simulink model "simple"  (R2020b)
settings: Solver=VariableStepAuto  StartTime=0.0  StopTime=Tf  RelTol=1e-3
values from neighbouring files (symbols this model uses):
  map = binaryOccupancyMap(maze, res)    [Run_Sim_LC.m]    (also in lidarPlanner.m = binaryOccupancyMap(                 [mapXLimits(2)-mapXLimit)
  N = size(waypoints, 1)    [interpolate_leg_waypoints.m]
  startPose = [2 2 0]    [Run_Sim_LC.m]
  Ts = 0.01    [Run_Sim_LC.m]
  waypoints = zeros(N, 4)    [get_leg_waypoints.m]    (also in leg_waypoints.m = linspace(start_config, goal_config, N); lidarPlanner.m = refpath.States(:,1:2))
undefined symbols (not defined in the file or in its folder): Discrete, Time, X, Y, Z
libraries: sm_lib x12, nesl_utility x3, hexapod x2, robotics_pg_exp_pack x2, ctrlSharedLib x1, robotalgslib x1
settings Model: Creator=fciriell  LastModifiedBy=zach
settings ExplorerConfigSet: InternalSimMechanicsExplorerSettings="<ExplorerConfiguration><canonicalview>default</canonicalview><AnimationSetting><BasePlaybackSpeed>1.0</BasePlaybackSpeed><PlaybackSpeedFactor>1.0</PlaybackSpeedFactor></AnimationSetting><TilePanel><TileInfo><Tiles Columns=\"1\" Count=\"2\" Rows=\"2\"><Column Weight=\"1\"/><Row Weight=\"0.4993\"/><Row Weight=\"0.5007\"/><Tile Height=\"1\" Width=\"1\" X=\"0\" Y=\"0\"/><Tile Height=\"1\" Width=\"1\" X=\"0\" Y=\"1\"/></Tiles></TileInfo><SceneInfo><SceneViewer><BGColor><R>1</R><G>1</G><B>1</B></BGColor><Camera><DoPerspective>on</DoPerspective><Position><X>-4.35147948962821829e-06</X><Y>-4.89869399804638128</Y><Z>0.176731420553238427</Z></Position><Center><X>-4.35147948962821829e-06</X><Y>-1.26250265135058726</Y><Z>0.176731420553238427</Z></Center><Up><X>0</X><Y>-0</Y><Z>1</Z></Up><ViewLimDist>1</ViewLimDist><YLim>0.466307658154998583</YLim><XLim>1.59125758717581123</XLim></Camera></SceneViewer><SceneViewer><BGColor><R>1</R><G>1</G><B>1</B></BGColor><Camera><DoPerspective>off</DoPerspective><Position><X>-5.9945065800093289e-08</X><Y>-3.21515629578642415</Y><Z>0.0606596897011122405</Z></Position><Center><X>-5.9945065800093289e-08</X><Y>-1.26250000733898382</Y><Z>0.0606596897011122405</Z></Center><Up><X>-0</X><Y>0</Y><Z>1</Z></Up><ViewLimDist>1</ViewLimDist><YLim>0.993270539045333911</YLim><XLim>3.37947076894122489</XLim></Camera></SceneViewer></SceneInfo></TilePanel><MechEditorPanel><Cameras><Camera><Id>Camera1</Id><Value><Name>Camera1</Name><NativeCamera><PositionTrackingFeature>camera.F</PositionTrackingFeature><CenterTrackingFeature>One_link_chain_dynamic.to_WF</CenterTrackingFeature><UpVectorTrackingFeature>camera.F</UpVectorTrackingFeature><CenterTrackingOrigin>on</CenterTrackingOrigin><UpVectorTrackingDirection>+Z</UpVectorTrackingDirection></NativeCamera></Value></Camera></Cameras><GfxPanelCameraMap><MapElement CameraMLId=\"Camera1\" GfxPanelIndex=\"0\"/></GfxPanelCameraMap><VideoCreator><PlaybackSpeedRatio>1.0</PlaybackSpeedRatio><FrameRate>30</FrameRate><VideoFormat>Motion JPEG AVI</VideoFormat><FrameSize>auto</FrameSize></VideoCreator></MechEditorPanel></ExplorerConfiguration>"

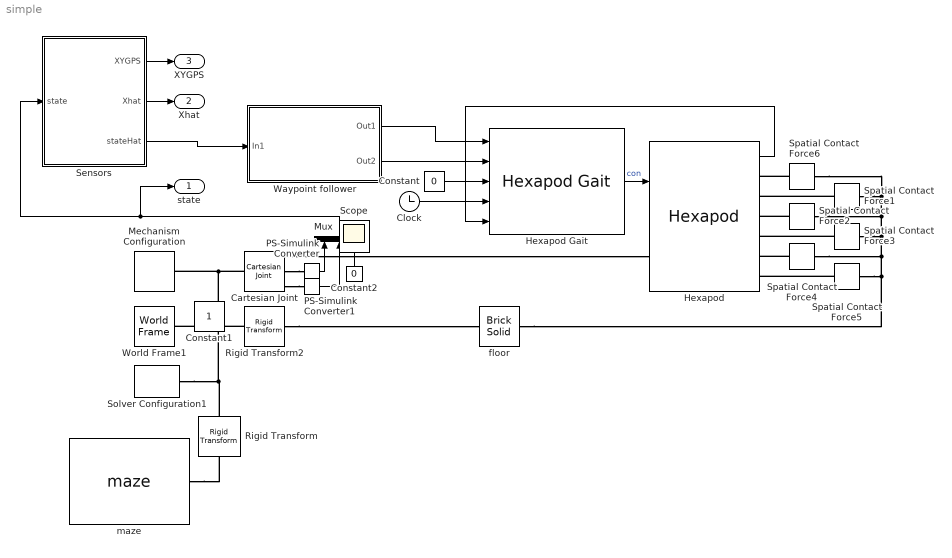
== system simple ==
  Cartesian Joint : sm_lib/Joints/Cartesian Joint  JointMode=Normal  SenseConstraintForce=off  SenseConstraintForceX=off  SenseConstraintForceY=off  SenseConstraintForceZ=off  SenseConstraintTorque=off  SenseConstraintTorqueX=off  SenseConstraintTorqueY=off  SenseConstraintTorqueZ=off  SenseTotalForce=off  SenseTotalForceX=off  SenseTotalForceY=off  SenseTotalForceZ=off  SenseTotalTorque=off  SenseTotalTorqueX=off  SenseTotalTorqueY=off  SenseTotalTorqueZ=off  CompositeWrenchDir=FollowerOnBase  CompositeWrenchFrame=BaseFrame  PxEquilibriumPosition=0  PxEquilibriumPositionUnits=m  PxSpringStiffness=0  PxSpringStiffnessUnits=N/m  PxDampingCoefficient=0  PxDampingCoefficientUnits=N/(m/s)  PxTorqueActuationMode=NoTorque  PxMotionActuationMode=ComputedMotion  PxSensePosition=on  PxSenseVelocity=off  PxSenseAcceleration=off  PxSenseTorqueForce=off  PxSenseLowerLimitTorqueForce=off  PxSenseUpperLimitTorqueForce=off  PxLowerLimitSpecify=off  PxLowerLimitBound=-1  PxLowerLimitBoundUnits=m  PxLowerLimitStiffness=1e6  PxLowerLimitStiffnessUnits=N/m  PxLowerLimitDamping=1e3  PxLowerLimitDampingUnits=N/(m/s)  PxLowerLimitTransitionRegionWidth=1e-4  PxLowerLimitTransitionRegionWidthUnits=m  PxUpperLimitSpecify=off  PxUpperLimitBound=1  PxUpperLimitBoundUnits=m  PxUpperLimitStiffness=1e6  PxUpperLimitStiffnessUnits=N/m  PxUpperLimitDamping=1e3  PxUpperLimitDampingUnits=N/(m/s)  PxUpperLimitTransitionRegionWidth=1e-4  PxUpperLimitTransitionRegionWidthUnits=m  PxPositionTargetSpecify=on  PxPositionTargetPriority=High  PxPositionTargetValue=startPose(1)  PxPositionTargetValueUnits=m  PxVelocityTargetSpecify=off  PxVelocityTargetPriority=High  PxVelocityTargetValue=0  PxVelocityTargetValueUnits=m/s  PyEquilibriumPosition=0  PyEquilibriumPositionUnits=m  PySpringStiffness=0  PySpringStiffnessUnits=N/m  PyDampingCoefficient=0  PyDampingCoefficientUnits=N/(m/s)  PyTorqueActuationMode=NoTorque  PyMotionActuationMode=ComputedMotion  PySensePosition=on  PySenseVelocity=off  PySenseAcceleration=off  PySenseTorqueForce=off  PySenseLowerLimitTorqueForce=off  PySenseUpperLimitTorqueForce=off  PyLowerLimitSpecify=off  PyLowerLimitBound=-1  PyLowerLimitBoundUnits=m  PyLowerLimitStiffness=1e6  PyLowerLimitStiffnessUnits=N/m  PyLowerLimitDamping=1e3  PyLowerLimitDampingUnits=N/(m/s)  PyLowerLimitTransitionRegionWidth=1e-4  PyLowerLimitTransitionRegionWidthUnits=m  PyUpperLimitSpecify=off  PyUpperLimitBound=1  PyUpperLimitBoundUnits=m  PyUpperLimitStiffness=1e6  PyUpperLimitStiffnessUnits=N/m  PyUpperLimitDamping=1e3  PyUpperLimitDampingUnits=N/(m/s)  PyUpperLimitTransitionRegionWidth=1e-4  PyUpperLimitTransitionRegionWidthUnits=m  PyPositionTargetSpecify=on  PyPositionTargetPriority=High  PyPositionTargetValue=startPose(2)  PyPositionTargetValueUnits=m  PyVelocityTargetSpecify=off  PyVelocityTargetPriority=High  PyVelocityTargetValue=0  PyVelocityTargetValueUnits=m/s  PzEquilibriumPosition=0  PzEquilibriumPositionUnits=m  PzSpringStiffness=0  PzSpringStiffnessUnits=N/m  PzDampingCoefficient=0  PzDampingCoefficientUnits=N/(m/s)  PzTorqueActuationMode=NoTorque  PzMotionActuationMode=ComputedMotion  PzSensePosition=off  PzSenseVelocity=off  PzSenseAcceleration=off  PzSenseTorqueForce=off  PzSenseLowerLimitTorqueForce=off  PzSenseUpperLimitTorqueForce=off  PzLowerLimitSpecify=off  PzLowerLimitBound=-1  PzLowerLimitBoundUnits=m  PzLowerLimitStiffness=1e6  PzLowerLimitStiffnessUnits=N/m  PzLowerLimitDamping=1e3  PzLowerLimitDampingUnits=N/(m/s)  PzLowerLimitTransitionRegionWidth=1e-4  PzLowerLimitTransitionRegionWidthUnits=m  PzUpperLimitSpecify=off  PzUpperLimitBound=1  PzUpperLimitBoundUnits=m  PzUpperLimitStiffness=1e6  PzUpperLimitStiffnessUnits=N/m  PzUpperLimitDamping=1e3  PzUpperLimitDampingUnits=N/(m/s)  PzUpperLimitTransitionRegionWidth=1e-4  PzUpperLimitTransitionRegionWidthUnits=m  PzPositionTargetSpecify=on  PzPositionTargetPriority=High  PzPositionTargetValue=0.35  PzPositionTargetValueUnits=m  PzVelocityTargetSpecify=off  PzVelocityTargetPriority=High  PzVelocityTargetValue=0  PzVelocityTargetValueUnits=m/s
  Clock : Clock
  Constant : Constant  Value=0  SampleTime=-1
  Constant2 : Constant  Value=0
  Hexapod : hexapod/Hexapod  leg_initial_config=[0; -pi/8; 5*pi/8]  leg_length_1=0.1  leg_length_2=0.4  leg_length_3=0.4  leg_radius=0.04  leg_mass_1=0.1  leg_mass_2=0.3  leg_mass_3=0.3  pos_kp=[80; 80; 80]  pos_ki=[0; 0; 0]  pos_kd=[10; 10; 10]  body_radius=0.3  body_mass=0.2
  Hexapod Gait : hexapod/Hexapod Gait  beta=0.55  T=0.6  contact_start_config=[0; -pi/8; 5*pi/8]  lifted_mid_theta2=-pi/4  lifted_mid_theta3=3*pi/4  body_radius=0.3  leg_length_1=0.1  leg_length_2=0.4  leg_length_3=0.4
  Mechanism Configuration : sm_lib/Utilities/Mechanism Configuration  UniformGravity=Constant  GravityVector=[0 0 -9.80665]  GravityVectorUnits=m/s^2  GravityUnits=m/s^2  LinearizationDelta=0.001  JointModeTransitionNonlinearIterations=2
  Mux : Mux  Inputs=3
  PS-Simulink Converter : nesl_utility/PS-Simulink Converter  PhysicalDomain=network_engine_domain  SubClassName=ps_output  LeftPortType=input  RightPortType=output  PseudoPeriodic=off  Frequencies=[]  Unit=inherit  AffineConversion=off
  PS-Simulink Converter1 : nesl_utility/PS-Simulink Converter  PhysicalDomain=network_engine_domain  SubClassName=ps_output  LeftPortType=input  RightPortType=output  PseudoPeriodic=off  Frequencies=[]  Unit=inherit  AffineConversion=off
  Rigid Transform : sm_lib/Frames and Transforms/Rigid Transform  TranslationMethod=StandardAxis  TranslationStandardOffset=0.01  TranslationLengthUnit=m  TranslationStandardAxis=-Z  TranslationCartesianOffset=[0 0 0]  TranslationROffset=0  TranslationROffsetUnits=m  TranslationZOffset=0  TranslationZOffsetUnits=m  TranslationThetaOffset=0  TranslationThetaOffsetUnits=deg  RotationMethod=None  RotationAngleUnits=deg  RotationStandardAxis=+Z  RotationAngle=0.0  RotationArbitraryAxis=[0 0 1]  FollAlignAxisA=+X  BaseAlignAxisA=+Y  FollAlignAxisB=+Y  BaseAlignAxisB=+Z  RotationSequenceAxes=FollowerAxes  RotationSequence=XYX  RotationSequenceAngles=[0 0 0]  RotationSequenceAnglesUnits=deg  RotationMatrix=[1 0 0; 0 1 0; 0 0 1]
  Rigid Transform2 : sm_lib/Frames and Transforms/Rigid Transform  TranslationMethod=Cartesian  TranslationStandardOffset=0  TranslationLengthUnit=m  TranslationStandardAxis=+Z  TranslationCartesianOffset=[(map.XWorldLimits(1)+map.XWorldLimits(2))/2 (map.YWorldLimits(1)+map.YWorldLimits(2))/2 0]  TranslationROffset=0  TranslationROffsetUnits=m  TranslationZOffset=0  TranslationZOffsetUnits=m  TranslationThetaOffset=0  TranslationThetaOffsetUnits=deg  RotationMethod=None  RotationAngleUnits=deg  RotationStandardAxis=+Z  RotationAngle=0.0  RotationArbitraryAxis=[0 0 1]  FollAlignAxisA=+X  BaseAlignAxisA=+Y  FollAlignAxisB=+Y  BaseAlignAxisB=+Z  RotationSequenceAxes=FollowerAxes  RotationSequence=XYX  RotationSequenceAngles=[0 0 0]  RotationSequenceAnglesUnits=deg  RotationMatrix=[1 0 0; 0 1 0; 0 0 1]
  Sensors : Subsystem
  Solver Configuration1 : nesl_utility/Solver Configuration  PhysicalDomain=network_engine_domain  SubClassName=solver  LeftPortType=input  RightPortType=generic  Tones=[]  Harmonics=[]  SimulateNoise=off  Profile=off  UseLocalSampling=off  EnableSwitchedLinearOptims=on  FrequencyDomain=off  UseCCode=off  RelTol=0.001  AbsTol=1e-06  MinStep=1e-09  ToWorkspace=off  RevertToSquareIcSolve=off  NumHomotopyIterations=100  PhasorMode=off  PhasorModeNumHarmonics=1  DoDC=off  ResidualTolerance=1e-09  UseLocalSolver=off  LocalSolverChoice=NE_BACKWARD_EULER_ADVANCER  LocalSolverSampleTime=0.001  DoFixedCost=off  MaxNonlinIter=3  MaxModeIter=2  ComputeImpulses=off  ImpulseIterations=2  LinearAlgebra=auto  EquationFormulation=NE_TIME_EF  DelaysMemoryBudget=1024  AutomaticFiltering=on  FilteringTimeConstant=0.001  PartitionStorageMethod=AS_NEEDED  PartitionMemoryBudget=1024  PartitionMethod=ROBUST
  Spatial Contact Force{1..6} (6 alike) : sm_lib/Forces and Torques/Spatial Contact Force  CoefficientOfDynamicFriction=0.3  CoefficientOfStaticFriction=0.9  NormalDamping=1e3  NormalDampingUnits=N/(m/s)  NormalStiffness=1e6  NormalStiffnessUnits=N/m  FrictionalCriticalVelocity=1e-3  FrictionalCriticalVelocityUnits=m/s  ZeroCrossDetectContactStartAndEnd=off  SenseFrictionalForceMagnitude=off  SenseNormalForceMagnitude=off  SenseSeparationDistance=off  NormalTransitionRegionWidth=1e-4  NormalTransitionRegionWidthUnits=m  FrictionType=SmoothStickSlip
  Waypoint follower : Subsystem
  World Frame1 : sm_lib/Frames and Transforms/World Frame
  floor : sm_lib/Body Elements/Brick Solid  GraphicAmbientColor=[0.15 0.15 0.15 1.0]  BasedOnType=Density  BrickDimensions=[(map.XWorldLimits(2)-map.XWorldLimits(1)) (map.YWorldLimits(2)-map.YWorldLimits(1)) 0.5]  BrickDimensionUnits=m  CenterOfMass=[0 0 0]  CenterOfMassUnits=m  GraphicDiffuseColor=[0.5 0.5 0.5]  Density=1000  DensityUnits=kg/m^3  DoExposeReferenceFrame=off  GraphicEmissiveColor=[0.0 0.0 0.0 1.0]  ExportEntireGeometry=on  SerializedFrames=<Frames><Frame><Id>Frame1</Id><Value><Name>TF</Name><Origin><Source>GeometricFeature</Source><FeatureName>+z surface</FeatureName></Origin><PrimaryAxis><DefinedDirection>+Z</DefinedDirection><Source>ReferenceFrame</Source><SourceDirection>+Z</SourceDirection><FeatureName></FeatureName></PrimaryAxis><SecondaryAxis><DefinedDirection>+X</DefinedDirection><Source>ReferenceFrame</Source><SourceDirection>+X</SourceDirection><FeatureName></FeatureName></SecondaryAxis></Value></Frame></Frames>  MarkerShape=Sphere  MarkerSize=10  GraphicType=FromGeometry  InertiaType=CalculateFromGeometry  Mass=1  MassUnits=kg  MomentsOfInertia=[1 1 1]  MomentsOfInertiaUnits=kg*m^2  GraphicOpacity=0.5  ProductsOfInertia=[0 0 0]  ProductsOfInertiaUnits=kg*m^2  GraphicShininess=75  GraphicSpecularColor=[0.5 0.5 0.5 1.0]  GraphicVisPropType=SimpleVisualProperties
  maze : robotics_pg_exp_pack/Environments & Sensors/Simscape Multibody Environments/maze  map=maze  wall_height=0.5  resolution=res  branching=branching
      settings: SourceProductName=Robotics Playground Expansion Pack
  state : Outport
  Xhat : Outport  Port=2
  XYGPS : Outport  Port=3
  Constant1 : Constant  IOType=siggen
  Scope : Scope
  wires:
  Hexapod Gait/1 -> Hexapod/1  "con"
  Hexapod/1 -> Hexapod Gait/5
  Constant/1 -> Hexapod Gait/3
  Clock/1 -> Hexapod Gait/4
  Mux/1 -> state/1, Sensors/1(state)
  Sensors/1(XYGPS) -> XYGPS/1
  Sensors/2(Xhat) -> Xhat/1
  Sensors/3(stateHat) -> Waypoint follower/1(In1)
  Waypoint follower/1(Out1) -> Hexapod Gait/1
  Waypoint follower/2(Out2) -> Hexapod Gait/2
  PS-Simulink Converter1/1 -> Mux/2
  PS-Simulink Converter/1 -> Mux/1
  Constant2/1 -> Mux/3
  connections:
  Cartesian Joint/RConn1 -- Hexapod/LConn1
  floor/RConn1 -- Spatial Contact Force5/LConn1 -- Spatial Contact Force4/LConn1 -- Spatial Contact Force3/LConn1 -- Spatial Contact Force2/LConn1 -- Spatial Contact Force1/LConn1 -- Spatial Contact Force6/LConn1
  Spatial Contact Force6/RConn1 -- Hexapod/RConn1
  Spatial Contact Force1/RConn1 -- Hexapod/RConn2
  Spatial Contact Force3/RConn1 -- Hexapod/RConn4
  Spatial Contact Force5/RConn1 -- Hexapod/RConn6
  Spatial Contact Force4/RConn1 -- Hexapod/RConn5
  Spatial Contact Force2/RConn1 -- Hexapod/RConn3
  Rigid Transform2/RConn1 -- floor/LConn1
  Solver Configuration1/RConn1 -- Rigid Transform/LConn1 -- Rigid Transform2/LConn1 -- Cartesian Joint/LConn1 -- Mechanism Configuration/RConn1 -- World Frame1/RConn1
  maze/RConn1 -- Rigid Transform/RConn1
  Cartesian Joint/RConn2 -- PS-Simulink Converter/LConn1
  Cartesian Joint/RConn3 -- PS-Simulink Converter1/LConn1

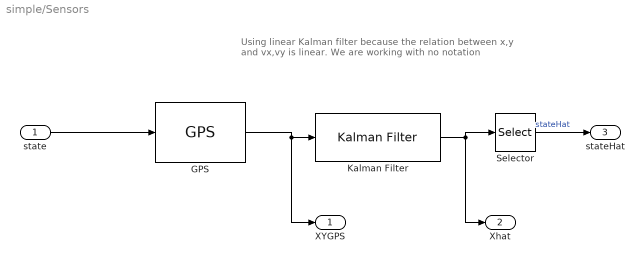
== system simple/Sensors ==
  note: Using linear Kalman filter because the relation between x,y and vx,vy is linear. We are working with no notation
  state : Inport
  "GPS " : robotics_pg_exp_pack/Environments & Sensors/GPS  xNoisePower=0.05  yNoisePower=0.05  Ts=Ts
      settings: SourceProductName=Robotics Playground Expansion Pack
  "Kalman Filter " : ctrlSharedLib/Kalman Filter  TimeDomain=Discrete-Time  UseCurrentEstimator=on  ModelSource=Individual A, B, C, D matrices  ModelSourceVariable=sys  A=[1 0 Ts 0; 0 1 0 Ts; 0 0 1 0; 0 0 0 1]  B=[0 0; 0 0; 1 0; 0 1]  C=[1 0 0 0; 0 1 0 0]  D=zeros(2)  NumberOfStates=2  NumberOfInputs=2  NumberOfOutputs=2  InitialEstimateSource=Dialog  X0=[startPose(1) startPose(2) 0 0]  P0=1e-3  UseK=off  UseGH=on  NumberOfProcessNoiseInputs=2  G=[Ts/2 0; 0 Ts/2; 1 0; 0 1]  TimeInvariantG=on  H=0  TimeInvariantH=on  Q=0.12  TimeInvariantQ=on  R=0.08  TimeInvariantR=on  N=0  TimeInvariantN=on  AddInputPort=off  AddEnablePort=off  OutputEstimatedY=off  OutputP=off  Ts=Ts
  Selector : Selector  InputPortWidth=4  IndexOptions=Index vector (dialog)  Indices=[1 2]  OutputSizes=1
  XYGPS : Outport
  Xhat : Outport  Port=2
  stateHat : Outport  Port=3
  wires:
  "GPS "/1 -> XYGPS/1, "Kalman Filter "/1
  Selector/1 -> stateHat/1  "stateHat"
  "Kalman Filter "/1 -> Selector/1, Xhat/1
  state/1 -> "GPS "/1

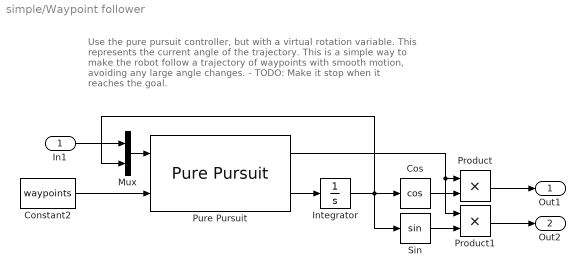
== system simple/Waypoint follower ==
  note: Use the pure pursuit controller, but with a virtual rotation variable.
      | This represents the current angle of the trajectory. This is a simple
      | way to make the robot follow a trajectory of waypoints with smooth
      | motion, avoiding any large angle changes.
      | - TODO: Make it stop when it reaches the goal.
  In1 : Inport
  Constant2 : Constant  Value=waypoints
  Cos : Trigonometry  Operator=cos
  Integrator : Integrator  InitialCondition=atan2(waypoints(2,2)-startPose(2), waypoints(1,2)-startPose(1))  WrapState=on
  Mux : Mux  Inputs=2
  Product : Product
  Product1 : Product
  Pure Pursuit : robotalgslib/Pure Pursuit  DesiredLinearVelocity=0.8  MaxAngularVelocity=3.14  LookaheadDistance=1.0  TargetDirPort=off  SimulateUsing=Code generation
  Sin : Trigonometry
  Out1 : Outport
  Out2 : Outport  Port=2
  wires:
  Integrator/1 -> Sin/1, Cos/1, Mux/2
  Constant2/1 -> Pure Pursuit/2
  Sin/1 -> Product1/2
  Pure Pursuit/2 -> Integrator/1
  In1/1 -> Mux/1
  Pure Pursuit/1 -> Product1/1, Product/1
  Cos/1 -> Product/2
  Mux/1 -> Pure Pursuit/1
  Product/1 -> Out1/1
  Product1/1 -> Out2/1
